simulink model "SymbSyncTemplate"  (R2022b)
settings: Solver=VariableStepAuto  StartTime=0.0  StopTime=0.2  RelTol=1e-3
model workspace (MAT data in the model file):
  f_b = 1000000
undefined symbols (not defined in the file or in its folder): comm, constellation
libraries: commfilt2 x3, commchan3 x1, dspsigops x1, commutil2 x1, commdigbbndpm3 x1, commsequence2 x1
settings Model: Creator=svdvl  LastModifiedBy=svdvl

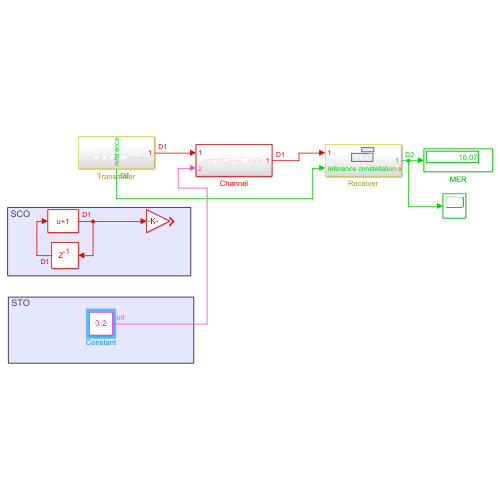
[thumbnail: Simulink's stored preview of the top-level diagram]
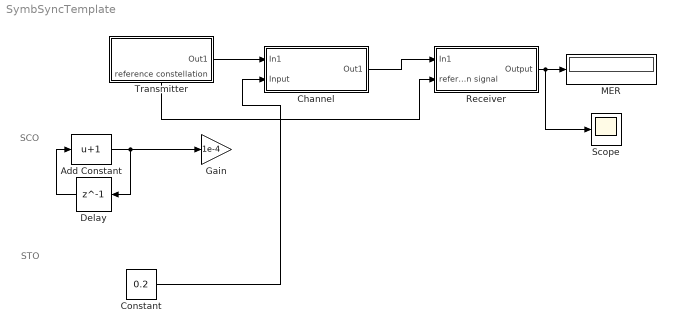
== system SymbSyncTemplate ==
  note: STO
  note: SCO
  Add Constant : Bias  Bias=1  SaturateOnIntegerOverflow=off
  Channel : Subsystem
  Constant : Constant  Value=0.2
  Delay : Delay  DelayLength=1  InitialCondition=0
  Gain : Gain  Gain=1e-4
  MER : Display
  Receiver : Subsystem
  Scope : Scope
  Transmitter : Subsystem
      settings: PortSchema="{\"entries\":[{\"content\":{\"sides\":[{\"content\":{\"connectorIds\":[]},\"type\":\"ConnectorPlacement.EquallySpacedRectSide\",\"uuid\":\"69c7c9c7-6fb5-4cca-8589-fbbeb91bac57\"},{\"content\":{\"connectorIds\":[\"Out1\"],\"side\":\"RIGHT\"},\"type\":\"ConnectorPlacement.EquallySpacedRectSide\",\"uuid\":\"39e38759-d35b-459b-8677-751191d3d25a\"},{\"content\":{\"connectorIds\":[],\"side\":\"TOP\"},\"type\":\"ConnectorPlacement.EquallySpacedRectSide\",\"uuid\":\"469cd50a-1b66-4166-9905-55abddab2769\"},{\"content\":{\"connectorIds\":[\"Out2\"],\"side\":\"BOTTOM\"},\"type\":\"ConnectorPlacement.EquallySpacedRectSide\",\"uuid\":\"3d50404d-9f80-49fe-a1b9-7d63ee4d6ab4\"}]},\"type\":\"ConnectorPlacement.EquallySpacedConnector\",\"uuid\":\"0722a572-8899-4bee-8b31-d1877a8c507f\"}],\"packageUris\":[\"http://schema.mathworks.com/mf0/Connector/R2020b\"],\"version\":\"1.0\"}"
  wires:
  Transmitter/1(Out1) -> Channel/1(In1)
  Channel/1(Out1) -> Receiver/1(In1)
  Add Constant/1 -> Gain/1, Delay/1
  Delay/1 -> Add Constant/1
  Receiver/1(Output) -> Scope/1, MER/1
  Transmitter/2(reference constellation) -> Receiver/2(reference constellation signal)
  Constant/1 -> Channel/2(Input)

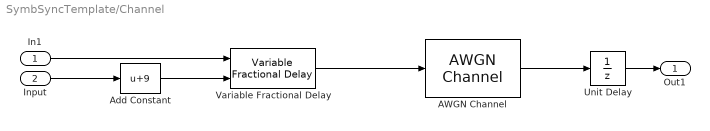
== system SymbSyncTemplate/Channel ==
  In1 : Inport
  Input : Inport  Port=2
  AWGN Channel : commchan3/AWGN Channel  InputProcessing=Columns as channels (frame based)  seed=67  noiseMode="Signal to noise ratio  (Es/No)"  EbNodB=10  EsNodB=20  SNRdB=10  bitsPerSym=1  Ps=1  Tsym=1/f_b  variance=1
  Add Constant : Bias  Bias=9  SaturateOnIntegerOverflow=off
  Unit Delay : UnitDelay  SampleTime=-1  HasFrameUpgradeWarning=on
  Variable Fractional Delay : dspsigops/Variable Fractional Delay  mode=OBSOLETE  modeActive=Farrow  L=4  FarrowL=20  R=10  alpha=1  dmax=2500  InputProcessing=Columns as channels (frame based)  ic=0  noDFT=off  fallbackFIR=Clip to the minimum value necessary for centered kernel  fallbackFarrow=Clip to the minimum value necessary for centered kernel  roundingMode=Zero  overflowMode=off
  Out1 : Outport
  wires:
  In1/1 -> Variable Fractional Delay/1
  AWGN Channel/1 -> Unit Delay/1
  Variable Fractional Delay/1 -> AWGN Channel/1
  Input/1 -> Add Constant/1
  Unit Delay/1 -> Out1/1
  Add Constant/1 -> Variable Fractional Delay/2

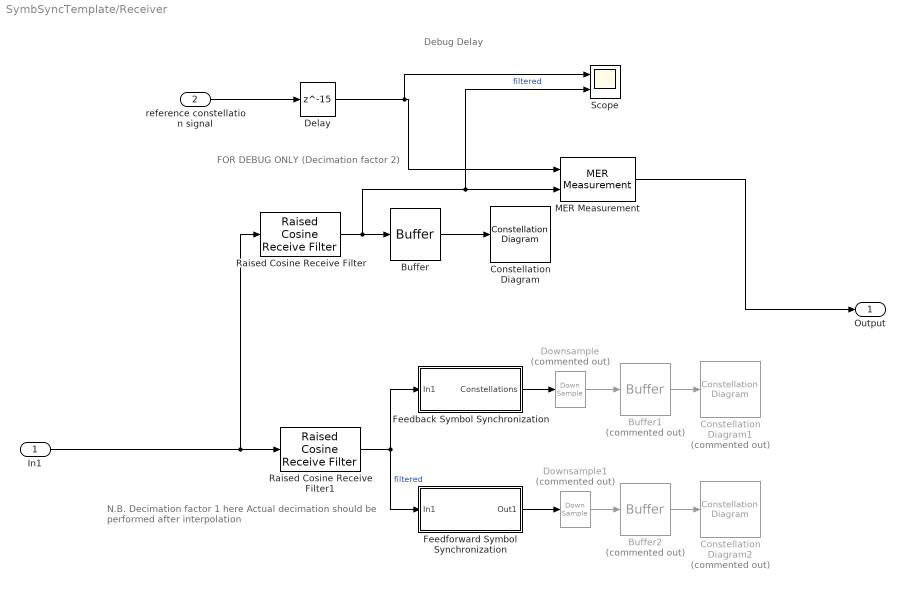
== system SymbSyncTemplate/Receiver ==
  note: Debug Delay
  note: N.B. Decimation factor 1 here
      | Actual decimation should be performed after interpolation
  note: FOR DEBUG ONLY (Decimation factor 2)
  In1 : Inport
  reference constellation signal : Inport  Port=2
  Buffer : Buffer  N=500  OutputFrames=off
  Buffer1 : Buffer  Commented=on  N=500  OutputFrames=off
  Buffer2 : Buffer  Commented=on  N=500  OutputFrames=off
  Constellation Diagram : ConstellationDiagram  WindowPosition=[382.000000,84.000000,600.000000,600.000000,]  Visible=on  ScopeFrameLocation=window  DefaultConfigurationName=comm.scopes.ConstellationDiagramBlockCfg
  Constellation Diagram1 : ConstellationDiagram  Commented=on  ScopeFrameLocation=window  DefaultConfigurationName=comm.scopes.ConstellationDiagramBlockCfg
  Constellation Diagram2 : ConstellationDiagram  Commented=on  ScopeFrameLocation=window  DefaultConfigurationName=comm.scopes.ConstellationDiagramBlockCfg
  Delay : Delay  DelayLength=15
  Downsample : DownSample  Commented=on
  Downsample1 : DownSample  Commented=on
  Feedback Symbol Synchronization : Subsystem
  Feedforward Symbol Synchronization : Subsystem
  MER Measurement : commutil2/MER Measurement  ReferenceSignalSource=Input port  ReferenceConstellation=constellation( comm.QPSKModulator )  MeasurementIntervalSource=Custom  MeasurementInterval=500  AveragingDimensions=1  MinimumMEROutputPort=off  XPercentileMEROutputPort=off  XPercentileValue=95  SymbolCountOutputPort=off  SimulateUsing=Interpreted execution
  Raised Cosine Receive Filter : commfilt2/Raised Cosine Receive Filter  filtType=Square root  R=0.5  filtSpan=10  N=2  downFactor=2  downOffset=0  filterGain=1  RateOptions=Allow multirate processing  framing=Mute  checkCoeff=off  variableName=rcRxFilt  currentFiltSpan=10  D=5  inputOffset=0  sampMode=Mute  saveAsFlag=0  rateMode=Downsampling  checkGain=Normalized  launchFVT=on  roundingMode=Floor  overflowMode=off  coeffDataTypeStr=Inherit: Same word length as input  coeffMin=[]  coeffMax=[]  coeffLastDataTypeStr=Inherit: Same word length as input  accumDataTypeStr=Inherit: Same as product output  accumLastDataTypeStr=Inherit: Same as product output  outputDataTypeStr=Inherit: Same as accumulator  outputMin=[]  outputMax=[]  outputLastDataTypeStr=Inherit: Same as accumulator
  Raised Cosine Receive Filter1 : commfilt2/Raised Cosine Receive Filter  filtType=Square root  R=0.5  filtSpan=10  N=2  downFactor=1  downOffset=0  filterGain=1  RateOptions=Allow multirate processing  framing=Mute  checkCoeff=off  variableName=rcRxFilt1  currentFiltSpan=10  D=5  inputOffset=0  sampMode=Mute  saveAsFlag=0  rateMode=Downsampling  checkGain=Normalized  launchFVT=on  roundingMode=Floor  overflowMode=off  coeffDataTypeStr=Inherit: Same word length as input  coeffMin=[]  coeffMax=[]  coeffLastDataTypeStr=Inherit: Same word length as input  accumDataTypeStr=Inherit: Same as product output  accumLastDataTypeStr=Inherit: Same as product output  outputDataTypeStr=Inherit: Same as accumulator  outputMin=[]  outputMax=[]  outputLastDataTypeStr=Inherit: Same as accumulator
  Scope : Scope  NumInputPorts=2
  Output : Outport
  wires:
  Raised Cosine Receive Filter/1 -> Scope/2, MER Measurement/2, Buffer/1  "filtered"
  Buffer/1 -> Constellation Diagram/1
  Raised Cosine Receive Filter1/1 -> Feedforward Symbol Synchronization/1(In1), Feedback Symbol Synchronization/1(In1)  "filtered"
  Feedback Symbol Synchronization/1(Constellations) -> Downsample/1
  Buffer1/1 -> Constellation Diagram1/1
  Feedforward Symbol Synchronization/1(Out1) -> Downsample1/1
  Buffer2/1 -> Constellation Diagram2/1
  MER Measurement/1 -> Output/1
  Downsample/1 -> Buffer1/1
  Downsample1/1 -> Buffer2/1
  reference constellation signal/1 -> Delay/1
  Delay/1 -> Scope/1, MER Measurement/1
  In1/1 -> Raised Cosine Receive Filter1/1, Raised Cosine Receive Filter/1

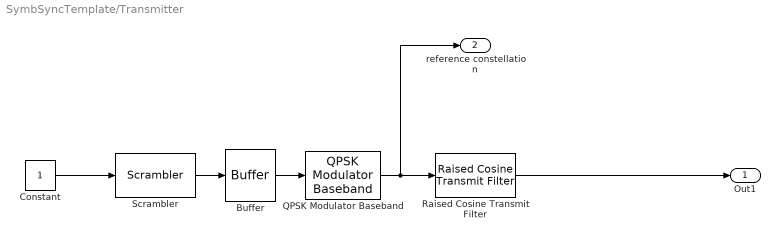
== system SymbSyncTemplate/Transmitter ==
  Buffer : Buffer  N=2  OutputFrames=off
  Constant : Constant  OutDataTypeStr=boolean  SampleTime=1/f_b
  QPSK Modulator Baseband : commdigbbndpm3/QPSK Modulator Baseband  InType=Bit  Enc=Gray  Ph=pi/4  outDtype=double  outWordLen=16  outUDDataType=sfix(16)  outFracLenMode=Best precision  outFracLen=15  outDataTypeStr=double  outLastDataTypeStr=double
  Raised Cosine Transmit Filter : commfilt2/Raised Cosine Transmit Filter  filtType=Square root  R=0.5  filtSpan=10  N=2  filterGain=1  RateOptions=Allow multirate processing  framing=Mute  checkCoeff=off  variableName=rcTxFilt1  checkGain=Normalized  sampMode=Mute  saveAsFlag=0  currentFiltSpan=10  D=5  launchFVT=on  roundingMode=Floor  overflowMode=off  coeffDataTypeStr=Inherit: Same word length as input  coeffMin=[]  coeffMax=[]  coeffLastDataTypeStr=Inherit: Same word length as input  outputDataTypeStr=Inherit: Same as accumulator  outputMin=[]  outputMax=[]  outputLastDataTypeStr=Inherit: Same as accumulator
  Scrambler : commsequence2/Scrambler  M=2  poly='1 + z^-1 + z^-2 + z^-4'  iniStaSource=Dialog Parameter  ini_sta=[0 1 0 0]  resetViaPort=off
  Out1 : Outport
  reference constellation : Outport  Port=2
  wires:
  QPSK Modulator Baseband/1 -> reference constellation/1, Raised Cosine Transmit Filter/1
  Raised Cosine Transmit Filter/1 -> Out1/1
  Scrambler/1 -> Buffer/1
  Constant/1 -> Scrambler/1
  Buffer/1 -> QPSK Modulator Baseband/1

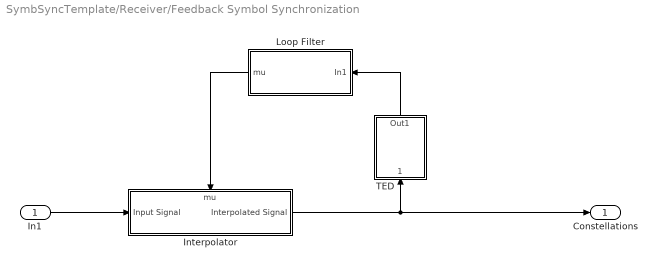
== system SymbSyncTemplate/Receiver/Feedback Symbol Synchronization ==
  In1 : Inport
  Interpolator : Subsystem
      settings: PortSchema="{\"entries\":[{\"content\":{\"sides\":[{\"content\":{\"connectorIds\":[\"In1\"]},\"type\":\"ConnectorPlacement.EquallySpacedRectSide\",\"uuid\":\"c7e0b39e-33d5-4eb5-b7d6-90764b5e62b8\"},{\"content\":{\"connectorIds\":[\"Out1\"],\"side\":\"RIGHT\"},\"type\":\"ConnectorPlacement.EquallySpacedRectSide\",\"uuid\":\"ac7422a2-3639-4236-b718-32242758d18a\"},{\"content\":{\"connectorIds\":[\"In2\"],\"side\":\"TOP\"},\"type\":\"ConnectorPlacement.EquallySpacedRectSide\",\"uuid\":\"6e9dd6c0-a168-4fc9-9763-85a1e572a310\"}]},\"type\":\"ConnectorPlacement.EquallySpacedConnector\",\"uuid\":\"22f84817-9463-46cb-a34b-0d92f7b44a53\"}],\"packageUris\":[\"http://schema.mathworks.com/mf0/Connector/R2020b\"],\"version\":\"1.0\"}"
  Loop Filter : Subsystem
  TED : Subsystem
  Constellations : Outport
  wires:
  In1/1 -> Interpolator/1(Input Signal)
  Loop Filter/1(mu) -> Interpolator/2(mu)
  TED/1(Out1) -> Loop Filter/1(In1)
  Interpolator/1(Interpolated Signal) -> Constellations/1, TED/1(Interpolated Signal)

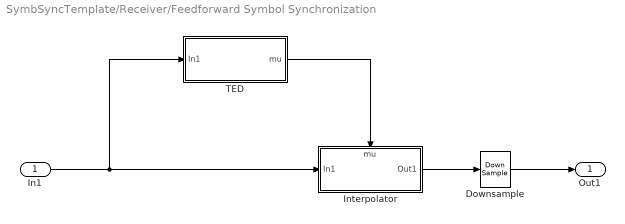
== system SymbSyncTemplate/Receiver/Feedforward Symbol Synchronization ==
  In1 : Inport
  Downsample : DownSample
  Interpolator : Subsystem
      settings: PortSchema="{\"entries\":[{\"content\":{\"sides\":[{\"content\":{\"connectorIds\":[\"In1\"]},\"type\":\"ConnectorPlacement.EquallySpacedRectSide\",\"uuid\":\"c7e0b39e-33d5-4eb5-b7d6-90764b5e62b8\"},{\"content\":{\"connectorIds\":[\"Out1\"],\"side\":\"RIGHT\"},\"type\":\"ConnectorPlacement.EquallySpacedRectSide\",\"uuid\":\"ac7422a2-3639-4236-b718-32242758d18a\"},{\"content\":{\"connectorIds\":[\"In2\"],\"side\":\"TOP\"},\"type\":\"ConnectorPlacement.EquallySpacedRectSide\",\"uuid\":\"6e9dd6c0-a168-4fc9-9763-85a1e572a310\"}]},\"type\":\"ConnectorPlacement.EquallySpacedConnector\",\"uuid\":\"22f84817-9463-46cb-a34b-0d92f7b44a53\"}],\"packageUris\":[\"http://schema.mathworks.com/mf0/Connector/R2020b\"],\"version\":\"1.0\"}"
  TED : Subsystem
  Out1 : Outport
  wires:
  Interpolator/1(Out1) -> Downsample/1
  In1/1 -> TED/1(In1), Interpolator/1(In1)
  TED/1(mu) -> Interpolator/2(mu)
  Downsample/1 -> Out1/1

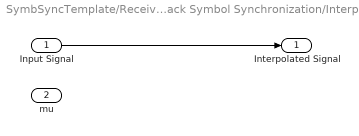
== system SymbSyncTemplate/Receiver/Feedback Symbol Synchronization/Interpolator ==
  Input Signal : Inport
  mu : Inport  Port=2
  Interpolated Signal : Outport
  wires:
  Input Signal/1 -> Interpolated Signal/1

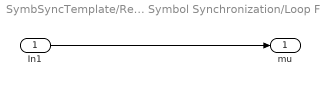
== system SymbSyncTemplate/Receiver/Feedback Symbol Synchronization/Loop Filter ==
  In1 : Inport
  mu : Outport
  wires:
  In1/1 -> mu/1

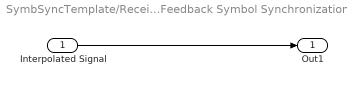
== system SymbSyncTemplate/Receiver/Feedback Symbol Synchronization/TED ==
  Interpolated Signal : Inport
  Out1 : Outport
  wires:
  Interpolated Signal/1 -> Out1/1

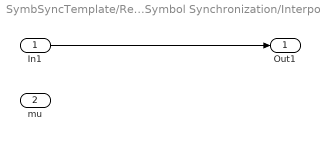
== system SymbSyncTemplate/Receiver/Feedforward Symbol Synchronization/Interpolator ==
  In1 : Inport
  mu : Inport  Port=2
  Out1 : Outport
  wires:
  In1/1 -> Out1/1

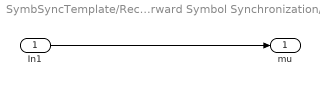
== system SymbSyncTemplate/Receiver/Feedforward Symbol Synchronization/TED ==
  In1 : Inport
  mu : Outport
  wires:
  In1/1 -> mu/1
